simulink model "LastWorkingModel"  (R2023b)
settings: Solver=FixedStepAuto  StartTime=0.0  StopTime=inf  FixedStep=0.01  RelTol=1e-3
values from neighbouring files (symbols this model uses):
  PWMBias = 35    [LQRJoe.m]    (also in LQRScript.m)
  PWMSat = 255    [LQRJoe.m]    (also in LQRScript.m)
  Reset = 0    [LQRJoe.m]
  uDist = 0    [LQRJoe.m]
  yDist = 0    [LQRJoe.m]
undefined symbols (not defined in the file or in its folder): K
libraries: simulink x2, arduinosensorlib x2, arduinolib x2
settings Model: ExtModeTrigDuration=2  Creator=M  LastModifiedBy=abdob
settings SolverCC: ConcurrentTasks=on  AlgebraicLoopSolver=TrustRegion  PositivePriorityOrder=on
settings OptimizationCC: BlockReduction=off  EnhancedBackFolding=on  PassReuseOutputArgsAs=Individual arguments  ZeroExternalMemoryAtStartup=off  ZeroInternalMemoryAtStartup=off  MaxStackSize=64  OptimizeBlockOrder=speed  DifferentSizesBufferReuse=on  OptimizationCustomize=off  EfficientTunableParamExpr=on
settings DebuggingCC: TasksWithSamePriorityMsg=none  ParameterTunabilityLossMsg=error  UnconnectedInputMsg=warning  UnconnectedOutputMsg=warning  UnconnectedLineMsg=warning
settings HardwareCC: ProdBitPerPointer=32  ProdBitPerSizeT=32  ProdBitPerPtrDiffT=32  ProdLargestAtomicInteger=Long  ProdLargestAtomicFloat=Double  ProdWordSize=32  ProdHWDeviceType=ARM Compatible->ARM Cortex
settings ModelReferenceCC: EnableRefExpFcnMdlSchedulingChecks=on
settings SFSimCC: MATLABDynamicMemAlloc=off
settings RTWCC: Description=Embedded Coder  SystemTargetFile=ert.tlc  HardwareBoard=ESP32-WROOM(Arduino Compatible)  TLCOptions="-aInlineSetEventsForThisBaseRateFcn=TLC_FALSE -aSuppressMultiTaskScheduler=TLC_FALSE  -aRateBasedStepFcn=0"  TemplateMakefile=ert_default_tmf  Toolchain=ESP32  BuildConfiguration=Faster Runs  CodeExecutionProfiling=on
settings CodeAppCC: ForceParamTrailComments=on  IgnoreCustomStorageClasses=off  OperatorAnnotations=on  SimulinkDataObjDesc=on  SFDataObjDesc=on  InsertBlockDesc=on
settings ERTTargetCC: TargetLangStandard=C99 (ISO)  SupportContinuousTime=on  SupportVariableSizeSignals=on  ExtModeTransport=3  ExtModeStaticAlloc=on  ExtModeAutomaticAllocSize=off  ExtModeStaticAllocSize=65536  ExtModeMexFile=ext_xcp  ExtModeIntrfLevel=Level2 - Open  RootIOFormat=Structure reference

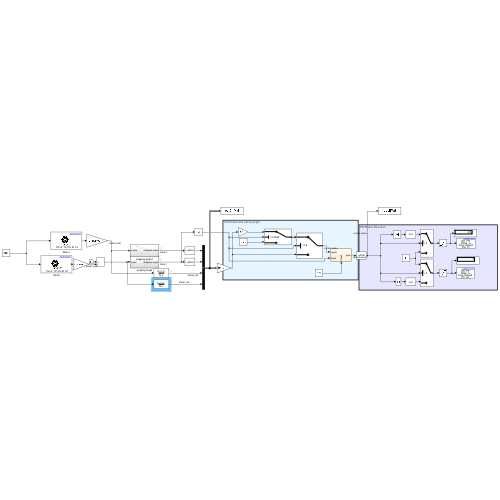
[thumbnail: Simulink's stored preview of the top-level diagram]
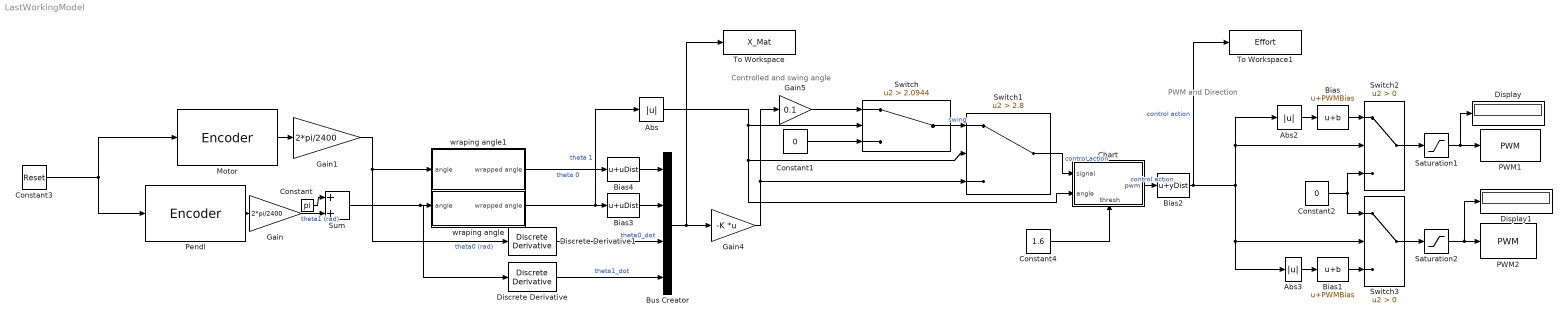
== system LastWorkingModel ==
  note: PWM and Direction
  note: Controlled and swing angle
  Abs : Abs  SaturateOnIntegerOverflow=off
  Abs2 : Abs  SaturateOnIntegerOverflow=off
  Abs3 : Abs  SaturateOnIntegerOverflow=off
  Bias : Bias  Bias=PWMBias  SaturateOnIntegerOverflow=off
  Bias1 : Bias  Bias=PWMBias  SaturateOnIntegerOverflow=off
  Bias2 : Bias  Bias=yDist  SaturateOnIntegerOverflow=off
  Bias3 : Bias  Bias=uDist  SaturateOnIntegerOverflow=off
  Bias4 : Bias  Bias=uDist  SaturateOnIntegerOverflow=off
  Bus Creator : BusCreator  Inputs=4
  Chart : Stateflow chart  TreatAsAtomicUnit=on
      settings: PortSchema="{\"entries\":[{\"content\":{\"sides\":[{\"content\":{\"connectorIds\":[\"In2\",\"In3\"]},\"type\":\"ConnectorPlacement.EquallySpacedRectSide\",\"uuid\":\"6fca160b-f029-4fe6-a24d-214834309ad8\"},{\"content\":{\"connectorIds\":[\"Out1\"],\"side\":\"RIGHT\"},\"type\":\"ConnectorPlacement.EquallySpacedRectSide\",\"uuid\":\"839f8058-e553-40ec-84a0-452c429905ec\"},{\"content\":{\"side\":\"TOP\"},\"type\":\"ConnectorPlacement.EquallySpacedRectSide\",\"uuid\":\"99673058-5cdf-40a6-9820-d742a9c4adea\"},{\"content\":{\"connectorIds\":[\"In1\"],\"side\":\"BOTTOM\"},\"type\":\"ConnectorPlacement.EquallySpacedRectSide\",\"uuid\":\"9d0e866b-39b0-4cce-be65-a605828b2662\"}]},\"type\":\"ConnectorPlacement.EquallySpacedConnector\",\"uuid\":\"30c7d6ac-9c3d-4d75-a9eb-59b3b85611f2\"}],\"packageUris\":[\"http://schema.mathworks.com/mf0/Connector/R2020b\"],\"version\":\"1.0\"}"
  Constant : Constant  Value=pi
  Constant1 : Constant  Value=0
  Constant2 : Constant  Value=0
  Constant3 : Constant  Value=Reset
  Constant4 : Constant  Value=1.6
  Discrete Derivative : simulink/Discrete/Discrete Derivative  gainval=1.0  ICPrevScaledInput=0.0  OutMin=[]  OutMax=[]  OutDataType=fixdt(1, 16)  OutScaling=2^-10  DoSatur=off
  Discrete Derivative1 : simulink/Discrete/Discrete Derivative  gainval=1.0  ICPrevScaledInput=0.0  OutMin=[]  OutMax=[]  OutDataType=fixdt(1, 16)  OutScaling=2^-10  DoSatur=off
  Display : Display
  Display1 : Display
  Gain : Gain  Gain=2*pi/2400  ParamDataTypeStr=double
  Gain1 : Gain  Gain=2*pi/2400  ParamDataTypeStr=double
  Gain4 : Gain  Gain=-K  Multiplication=Matrix(K*u) (u vector)
  Gain5 : Gain  Gain=0.1
  Motor : arduinosensorlib/Encoder  InputA=13  InputB=14  Mode=Reset by external signal  SampleTime=-1
  PWM1 : arduinolib/PWM  pinNumber=21  frequencyType=Default  desiredFrequency=200  achievableFrequency=200
  PWM2 : arduinolib/PWM  pinNumber=22  frequencyType=Default  desiredFrequency=200  achievableFrequency=200
  Pendl : arduinosensorlib/Encoder  InputA=19  InputB=18  Mode=Reset by external signal  SampleTime=-1
  Saturation1 : Saturate  UpperLimit=PWMSat  LowerLimit=0
  Saturation2 : Saturate  UpperLimit=PWMSat  LowerLimit=0
  Sum : Sum  Inputs=|++
  Switch : Switch  Criteria=u2 > Threshold  Threshold=2.0944  SaturateOnIntegerOverflow=off  InputSameDT=off
  Switch1 : Switch  Criteria=u2 > Threshold  Threshold=2.8  SaturateOnIntegerOverflow=off  InputSameDT=off
  Switch2 : Switch  Criteria=u2 > Threshold  SaturateOnIntegerOverflow=off  InputSameDT=off
  Switch3 : Switch  Criteria=u2 > Threshold  SaturateOnIntegerOverflow=off  InputSameDT=off
  To Workspace : ToWorkspace  VariableName=X_Mat  SaveFormat=Timeseries  SampleTime=-1
      settings: MaxDataPoints=500
  To Workspace1 : ToWorkspace  VariableName=Effort  SaveFormat=Timeseries  SampleTime=-1
  wraping angle : Subsystem
  wraping angle1 : Subsystem
  wires:
  Motor/1 -> Gain1/1
  Pendl/1 -> Gain/1
  Constant/1 -> Sum/1
  Gain/1 -> Sum/2  "theta1 (rad)"
  Sum/1 -> Discrete Derivative/1, wraping angle/1(angle)
  wraping angle/1(wrapped angle) -> Bias3/1, Abs/1  "theta 1"
  Abs/1 -> Chart/3(angle), Switch1/2, Switch/2
  Switch/1 -> Switch1/1  "swing"
  Constant1/1 -> Switch/3
  Gain5/1 -> Switch/1
  Saturation2/1 -> PWM2/1, Display1/1
  Gain4/1 -> Switch1/3, Gain5/1
  Discrete Derivative/1 -> Bus Creator/4  "theta1_dot"
  Discrete Derivative1/1 -> Bus Creator/3  "theta0_dot"
  Switch1/1 -> Chart/2(signal)  "control action"
  Bus Creator/1 -> To Workspace/1, Gain4/1
  Switch2/1 -> Saturation1/1
  Switch3/1 -> Saturation2/1
  Abs2/1 -> Bias/1
  Bias/1 -> Switch2/1
  Abs3/1 -> Bias1/1
  Bias1/1 -> Switch3/3
  Bias2/1 -> To Workspace1/1, Abs3/1, Switch3/2, Abs2/1, Switch2/2  "control action"
  Saturation1/1 -> PWM1/1, Display/1
  Constant2/1 -> Switch3/1, Switch2/3
  Gain1/1 -> Discrete Derivative1/1, wraping angle1/1(angle)  "theta0 (rad)"
  Constant3/1 -> Pendl/1, Motor/1
  Chart/1(pwm) -> Bias2/1  "control action"
  Bias3/1 -> Bus Creator/2
  wraping angle1/1(wrapped angle) -> Bias4/1  "theta 0"
  Bias4/1 -> Bus Creator/1
  Constant4/1 -> Chart/1(thresh)

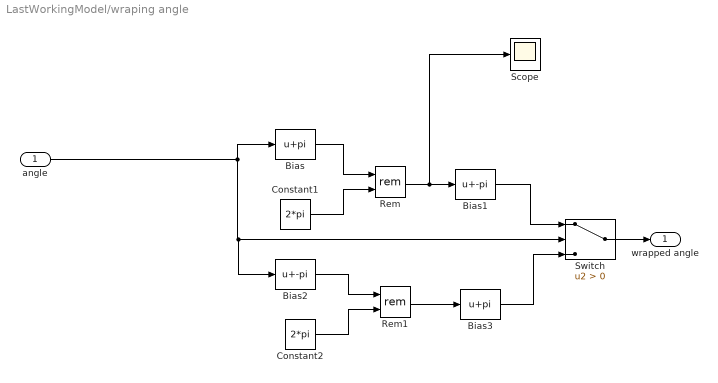
== system LastWorkingModel/wraping angle ==
  angle : Inport
  Bias : Bias  Bias=pi  SaturateOnIntegerOverflow=off
  Bias1 : Bias  Bias=-pi  SaturateOnIntegerOverflow=off
  Bias2 : Bias  Bias=-pi  SaturateOnIntegerOverflow=off
  Bias3 : Bias  Bias=pi  SaturateOnIntegerOverflow=off
  Constant1 : Constant  Value=2*pi
  Constant2 : Constant  Value=2*pi
  Rem : Math  Operator=rem
  Rem1 : Math  Operator=rem
  Scope : Scope
  Switch : Switch  Criteria=u2 > Threshold  SaturateOnIntegerOverflow=off  InputSameDT=off
  wrapped angle : Outport
  wires:
  Bias/1 -> Rem/1
  Rem1/1 -> Bias3/1
  Bias3/1 -> Switch/3
  Constant1/1 -> Rem/2
  Constant2/1 -> Rem1/2
  Bias1/1 -> Switch/1
  Bias2/1 -> Rem1/1
  Rem/1 -> Scope/1, Bias1/1
  Switch/1 -> wrapped angle/1
  angle/1 -> Bias/1, Bias2/1, Switch/2

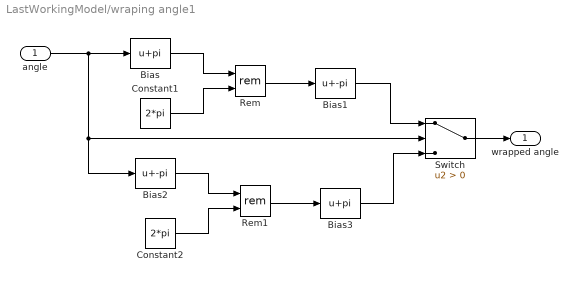
== system LastWorkingModel/wraping angle1 ==
  angle : Inport
  Bias : Bias  Bias=pi  SaturateOnIntegerOverflow=off
  Bias1 : Bias  Bias=-pi  SaturateOnIntegerOverflow=off
  Bias2 : Bias  Bias=-pi  SaturateOnIntegerOverflow=off
  Bias3 : Bias  Bias=pi  SaturateOnIntegerOverflow=off
  Constant1 : Constant  Value=2*pi
  Constant2 : Constant  Value=2*pi
  Rem : Math  Operator=rem
  Rem1 : Math  Operator=rem
  Switch : Switch  Criteria=u2 > Threshold  SaturateOnIntegerOverflow=off  InputSameDT=off
  wrapped angle : Outport
  wires:
  Switch/1 -> wrapped angle/1
  Rem/1 -> Bias1/1
  Bias2/1 -> Rem1/1
  Bias1/1 -> Switch/1
  Constant2/1 -> Rem1/2
  Constant1/1 -> Rem/2
  Bias3/1 -> Switch/3
  Rem1/1 -> Bias3/1
  angle/1 -> Bias/1, Bias2/1, Switch/2
  Bias/1 -> Rem/1

== stateflow chart LastWorkingModel/Chart ==
  note: %%angle < 135
  state start
    pwm = 255
  state stop
    pwm = signal
  (default) -> start
  start -> stop : [angle < (thresh)]
  stop -> start : [[ angle >(thresh)] && after(2,sec)]
  data: thresh input; signal input; angle input; pwm output
